simulink model "Project_lqr_control"  (R2025b)
settings: Solver=FixedStepDiscrete  StartTime=0.0  StopTime=inf  FixedStep=TS  RelTol=1e-3  EnableMultiTasking=on
values from neighbouring files (symbols this model uses):
  ES = -C2DEG*D2R    (= -0.00872664625997)    [NXT_Parameters.m]
  GS = GyroS*D2R    [NXT_Parameters.m]
  KLQR = [ 70.7107   73.7136 -108.1757  -16.8574]    [NXT_Parameters.m]    (also in Project_Jayce.m = lqr(A_b, B_b, Q, R))
  Rw = 0.021336    [NXT_Parameters.m]
  TS = 0.005    [NXT_Parameters.m]
libraries: arduinolib x3, simulink x1
settings Model: ExtModeTrigDuration=2  Creator=Sang  LastModifiedBy=jboar
settings SolverCC: AlgebraicLoopSolver=TrustRegion
settings DataIOCC: ReturnWorkspaceOutputs=off
settings OptimizationCC: MaxStackSize=64  EfficientTunableParamExpr=on
settings DebuggingCC: ParameterTunabilityLossMsg=error  UnconnectedInputMsg=warning  UnconnectedOutputMsg=warning  UnconnectedLineMsg=warning  ArithmeticOperatorsInVariantConditions=warning
settings HardwareCC: ProdBitPerInt=16.0  ProdBitPerPointer=16.0  ProdBitPerSizeT=16.0  ProdBitPerPtrDiffT=16.0  ProdLargestAtomicFloat=None  ProdWordSize=8.0  ProdHWDeviceType=Atmel->AVR
settings ModelReferenceCC: EnableRefExpFcnMdlSchedulingChecks=on
settings SFSimCC: SimUseLocalCustomCode=off  MATLABDynamicMemAlloc=off  CustomCodeUndefinedFunction=UseInterfaceOnly
settings RTWCC: SystemTargetFile=ert.tlc  HardwareBoard=Arduino Mega 2560  TemplateMakefile=ert_default_tmf  GenerateReport=on  RTWUseLocalCustomCode=off  Toolchain=Arduino AVR  BuildConfiguration=Faster Runs  IncludeHyperlinkInReport=on  LaunchReport=on  GenerateTraceInfo=on  GenerateTraceReport=on  GenerateTraceReportSl=on  GenerateTraceReportSf=on  GenerateTraceReportEml=on  GPUComputeCapability=3.5  Description=Embedded Coder
settings CodeAppCC: ForceParamTrailComments=on  IgnoreCustomStorageClasses=off  OperatorAnnotations=on  SimulinkDataObjDesc=on  SFDataObjDesc=on  MATLABFcnDesc=on  InsertBlockDesc=on  StateflowObjectComments=on  MATLABSourceComments=on
settings ERTTargetCC: InlinedParameterPlacement=Hierarchical  DynamicArrayContainerType=coder::array  MultiwordLength=2048.0  SupportContinuousTime=on  SupportVariableSizeSignals=on

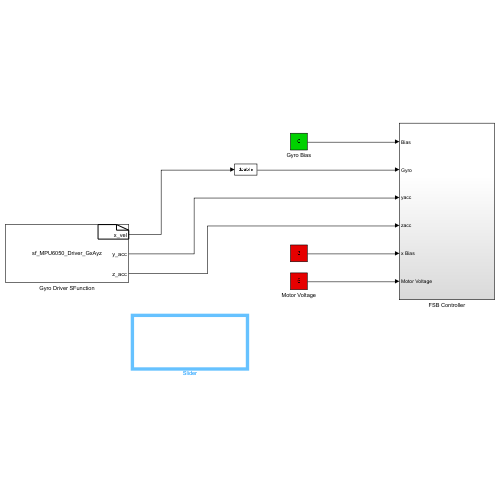
[thumbnail: Simulink's stored preview of the top-level diagram]
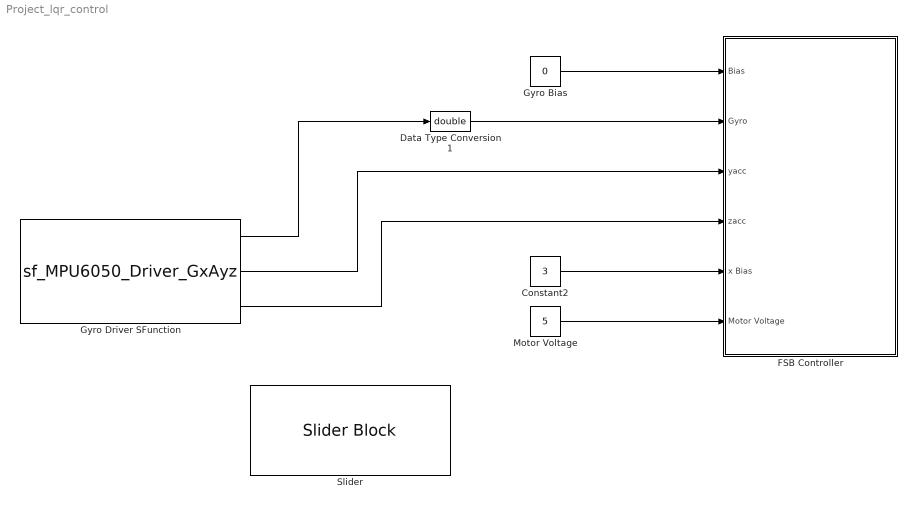
== system Project_lqr_control ==
  Constant2 : Constant  Value=3
  Data Type Conversion1 : DataTypeConversion  OutDataTypeStr=double  SaturateOnIntegerOverflow=off  RndMeth=Floor
  FSB Controller : Subsystem
  Gyro Bias : Constant  Value=0
  Gyro Driver SFunction : S-Function  InitFcn=try, set_param(gcb,'FunctionName','sf_MPU6050_Driver_GxAyz'), end  FunctionName=sf_MPU6050_Driver_GxAyz  SFunctionModules=sf_MPU6050_Driver_GxAyz_wrapper.cpp  SFunctionDeploymentMode=off  EnableBusSupport=off  mask(S-Function Builder){}
      mask help: Simulink:masks:SFunctionBuilder_MD
      mask init:
      | val = [[.9  0.75 0.75 1 1 .9 .9 1]',[1 1 0.75 0.75 .9 .9 1 .9]'];try , sys = get_param(gcb,'SfunBuilderFcnName');if isempty(sys), sys = get_param(gcb,'FunctionName'); end,catch, sys = get_param(gcb,'FunctionName'); end
      settings: CopyFcn=set_param(gcbh,'LinkStatus','none')  PreSaveFcn=try, set_param(gcb,'FunctionName','sf_MPU6050_Driver_GxAyz'), end  OpenFcn=sfunctionwizard(gcbh)
      mask Display:
      | plot(val(:,1),val(:,2))
      | disp(sys)
      | port_label('output',1,sprintf('%s', 'x\_vel'),'interpreter','tex')
      | port_label('output',2,sprintf('%s', 'y\_acc'),'interpreter','tex')
      | port_label('output',3,sprintf('%s', 'z\_acc'),'interpreter','tex')
  Motor Voltage : Constant  Value=5
  Slider : SliderBlock  ScaleMin=-20  ScaleMax=20
  wires:
  Gyro Driver SFunction/2 -> FSB Controller/3("yacc ")
  Gyro Driver SFunction/3 -> FSB Controller/4("zacc ")
  Gyro Bias/1 -> FSB Controller/1(Bias)
  Constant2/1 -> FSB Controller/5(x Bias)
  Motor Voltage/1 -> FSB Controller/6(Motor Voltage)
  Gyro Driver SFunction/1 -> Data Type Conversion1/1
  Data Type Conversion1/1 -> FSB Controller/2(Gyro)

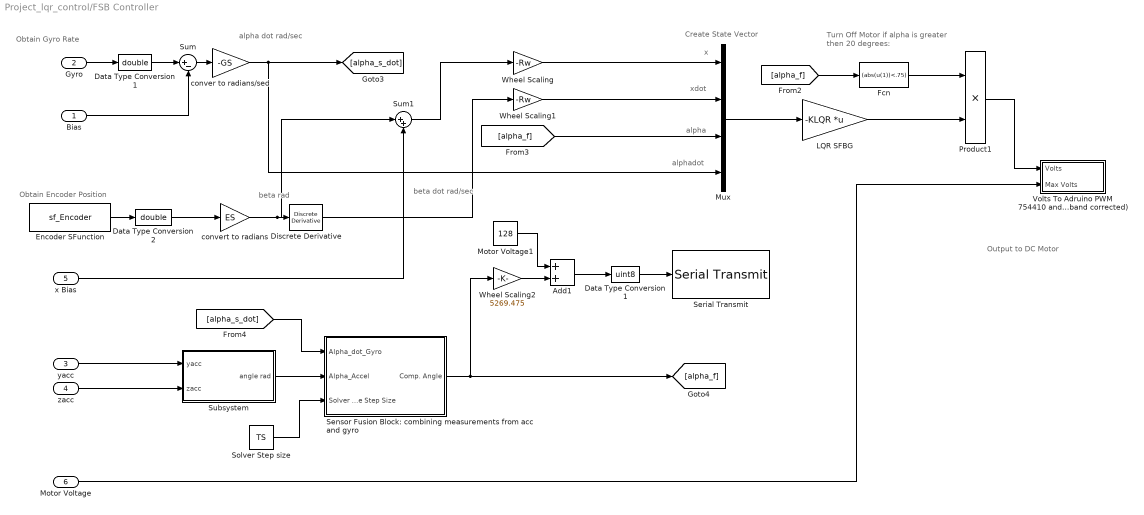
== system Project_lqr_control/FSB Controller ==
  note: Turn Off Motor if alpha is
      | greater then 20 degrees:
  note: Output to DC Motor
  note: Create State Vector
  note: Obtain Encoder Position
  note: Obtain Gyro Rate
  note: xdot
  note: x
  note: beta
      | rad
  note: alpha dot
      | rad/sec
  note: beta dot
      | rad/sec
  note: alpha
  note: alphadot
  Bias : Inport
  Gyro : Inport  Port=2
  "yacc " : Inport  Port=3
  "zacc " : Inport  Port=4
  x Bias : Inport  Port=5
  Motor Voltage : Inport  Port=6
  Add1 : Sum
  Data Type Conversion1 : DataTypeConversion  OutDataTypeStr=double  SaturateOnIntegerOverflow=off  RndMeth=Floor
  Data Type Conversion2 : DataTypeConversion  OutDataTypeStr=double  SaturateOnIntegerOverflow=off  RndMeth=Floor
  Data Type Conversion1 : DataTypeConversion  OutDataTypeStr=uint8  RndMeth=Nearest  SaturateOnIntegerOverflow=off
  Discrete Derivative : simulink/Discrete/Discrete Derivative  gainval=1.0  ICPrevScaledInput=0.0  OutMin=[]  OutMax=[]  OutDataType=fixdt(1, 16)  OutScaling=2^-10  DoSatur=off
  Encoder SFunction : S-Function  InitFcn=try, set_param(gcb,'FunctionName','sf_Encoder'), end  FunctionName=sf_Encoder  Parameters=uint8(0),uint8(18),uint8(19)  SFunctionModules=sf_Encoder_wrapper  SFunctionDeploymentMode=off  EnableBusSupport=off  mask(S-Function Builder){}
      mask init: same as Project_lqr_control/Gyro Driver SFunction
      settings: CopyFcn=set_param(gcbh,'LinkStatus','none')  PreSaveFcn=try, set_param(gcb,'FunctionName','sf_Encoder'), end  OpenFcn=sfunctionwizard(gcbh)
      mask Display: plot(val(:,1),val(:,2)),disp(sys), port_label('output',1,'pos')
  Fcn : Fcn  Expr=(abs(u(1))<.75)
  LQR SFBG : Gain  Gain=-KLQR  Multiplication=Matrix(K*u)
  Motor Voltage1 : Constant  Value=128
  Mux : Mux
  Product1 : Product  RndMeth=Zero
  Sensor Fusion Block: combining measurements from acc and gyro : Subsystem
  Serial Transmit : arduinolib/Serial Transmit  portNumber=2  sendmode=write  sendformat=Decimal  floatprecision=2  header=[]  terminator=[]  blockPlatform=arduino
  Solver Step size : Constant  Value=TS
  Subsystem : Subsystem
  Sum : Sum  Inputs=|+-
  Sum1 : Sum  Inputs=|++
  Volts To Adruino PWM 754410 and Motor1 (Deadband corrected) : Subsystem
  Wheel Scaling : Gain  Gain=-Rw
  Wheel Scaling1 : Gain  Gain=-Rw
  Wheel Scaling2 : Gain  Gain=5269.475
  conver to radians/sed : Gain  Gain=-GS
  convert to radians : Gain  Gain=ES  OutDataTypeStr=double
  wires:
  Bias/1 -> Sum/2
  Sum/1 -> conver to radians/sed/1
  convert to radians/1 -> Sum1/1, Discrete Derivative/1
  Data Type Conversion1/1 -> Sum/1
  Gyro/1 -> Data Type Conversion1/1
  [alpha_f] -> Fcn/1
  conver to radians/sed/1 -> [alpha_s_dot], Mux/4
  "yacc "/1 -> Subsystem/1(yacc)
  "zacc "/1 -> Subsystem/2(zacc)
  [alpha_f] -> Mux/3
  LQR SFBG/1 -> Product1/2
  Fcn/1 -> Product1/1
  Mux/1 -> LQR SFBG/1
  Wheel Scaling/1 -> Mux/1
  Subsystem/1(angle rad) -> Sensor Fusion Block: combining measurements from acc and gyro/2(Alpha_Accel)
  [alpha_s_dot] -> Sensor Fusion Block: combining measurements from acc and gyro/1(Alpha_dot_Gyro)
  Solver Step size/1 -> Sensor Fusion Block: combining measurements from acc and gyro/3(Solver Time Step Size)
  Sensor Fusion Block: combining measurements from acc and gyro/1(Comp. Angle) -> Wheel Scaling2/1, [alpha_f]
  Wheel Scaling1/1 -> Mux/2
  x Bias/1 -> Sum1/2
  Sum1/1 -> Wheel Scaling/1
  Encoder SFunction/1 -> Data Type Conversion2/1
  Data Type Conversion2/1 -> convert to radians/1
  Product1/1 -> Volts To Adruino PWM 754410 and Motor1 (Deadband corrected)/1(Volts)
  Motor Voltage/1 -> Volts To Adruino PWM 754410 and Motor1 (Deadband corrected)/2(Max Volts)
  Data Type Conversion1/1 -> Serial Transmit/1
  Add1/1 -> Data Type Conversion1/1
  Wheel Scaling2/1 -> Add1/2
  Motor Voltage1/1 -> Add1/1
  Discrete Derivative/1 -> Wheel Scaling1/1

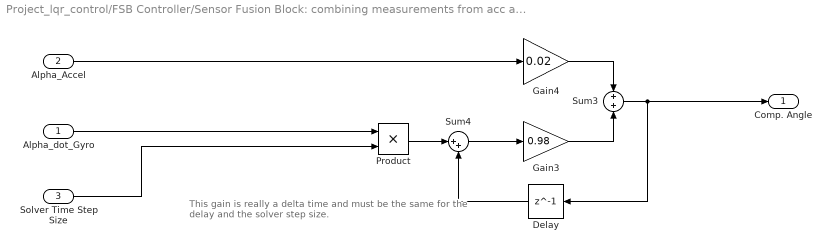
== system Project_lqr_control/FSB Controller/Sensor Fusion Block: combining measurements from acc and gyro ==
  note: This gain is really a delta time and must be the same for
      | the delay and the solver step size.
  Alpha_dot_Gyro : Inport
  Alpha_Accel : Inport  Port=2
  Solver Time Step Size : Inport  Port=3
  Delay : Delay  DelayLength=1  InitialCondition=0
  Gain3 : Gain  Gain=0.98
  Gain4 : Gain  Gain=0.02
  Product : Product
  Sum3 : Sum
  Sum4 : Sum  Inputs=|++
  Comp. Angle : Outport  VectorParamsAs1DForOutWhenUnconnected=off
  wires:
  Gain3/1 -> Sum3/2
  Gain4/1 -> Sum3/1
  Sum3/1 -> Comp. Angle/1, Delay/1
  Sum4/1 -> Gain3/1
  Delay/1 -> Sum4/2
  Product/1 -> Sum4/1
  Alpha_Accel/1 -> Gain4/1
  Alpha_dot_Gyro/1 -> Product/1
  Solver Time Step Size/1 -> Product/2

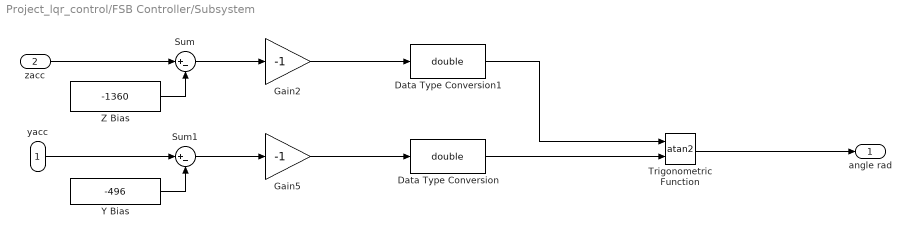
== system Project_lqr_control/FSB Controller/Subsystem ==
  yacc : Inport
  zacc : Inport  Port=2
  Data Type Conversion : DataTypeConversion  OutDataTypeStr=double  SaturateOnIntegerOverflow=off  RndMeth=Floor
  Data Type Conversion1 : DataTypeConversion  OutDataTypeStr=double  SaturateOnIntegerOverflow=off  RndMeth=Floor
  Gain2 : Gain  Gain=-1
  Gain5 : Gain  Gain=-1
  Sum : Sum  Inputs=|+-
  Sum1 : Sum  Inputs=|+-
  Trigonometric Function : Trigonometry  Operator=atan2
  Y Bias : Constant  Value=-496
  Z Bias : Constant  Value=-1360
  angle rad : Outport  VectorParamsAs1DForOutWhenUnconnected=off
  wires:
  Z Bias/1 -> Sum/2
  Y Bias/1 -> Sum1/2
  Trigonometric Function/1 -> angle rad/1
  Data Type Conversion1/1 -> Trigonometric Function/1
  Data Type Conversion/1 -> Trigonometric Function/2
  zacc/1 -> Sum/1
  yacc/1 -> Sum1/1
  Gain2/1 -> Data Type Conversion1/1
  Sum/1 -> Gain2/1
  Sum1/1 -> Gain5/1
  Gain5/1 -> Data Type Conversion/1

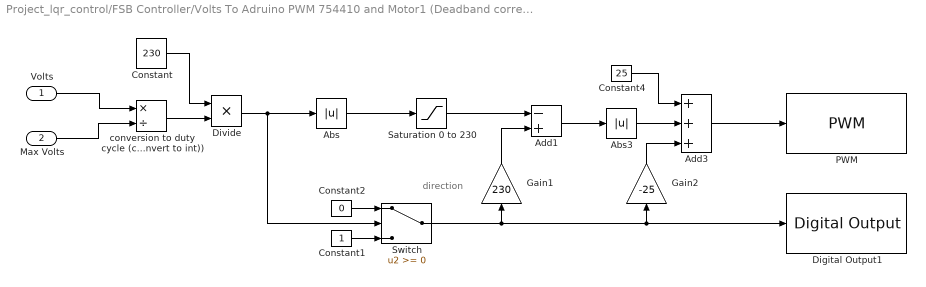
== system Project_lqr_control/FSB Controller/Volts To Adruino PWM 754410 and Motor1 (Deadband corrected) ==
  note: direction
  Volts : Inport
  Max Volts : Inport  Port=2
  Abs : Abs  SaturateOnIntegerOverflow=off
  Abs3 : Abs  SaturateOnIntegerOverflow=off
  Add1 : Sum  Inputs=-+
  Add3 : Sum  Inputs=+++
  Constant : Constant  Value=230
  Constant1 : Constant
  Constant2 : Constant  Value=0
  Constant4 : Constant  Value=25
  Digital Output1 : arduinolib/Digital Output  pinNumber=8  Direction=output  blockPlatform=arduino
  Divide : Product  Inputs=**
  Gain1 : Gain  Gain=230
  Gain2 : Gain  Gain=-25
  PWM : arduinolib/PWM  pinNumber=6  frequencyType=Default  desiredFrequency=490.2  achievableFrequency=490.2
  Saturation 0 to 230 : Saturate  UpperLimit=230  LowerLimit=0
  Switch : Switch  SaturateOnIntegerOverflow=off  InputSameDT=off
  conversion to duty cycle (convert to int)) : Product  Inputs=*/  OutDataTypeStr=double
  wires:
  Abs/1 -> Saturation 0 to 230/1
  Saturation 0 to 230/1 -> Add1/1
  Add1/1 -> Abs3/1
  Gain1/1 -> Add1/2
  Constant1/1 -> Switch/3
  Constant2/1 -> Switch/1
  Switch/1 -> Gain1/1, Gain2/1, Digital Output1/1
  Abs3/1 -> Add3/2
  Add3/1 -> PWM/1
  Constant4/1 -> Add3/1
  Volts/1 -> conversion to duty cycle (convert to int))/1
  Max Volts/1 -> conversion to duty cycle (convert to int))/2
  Divide/1 -> Switch/2, Abs/1
  conversion to duty cycle (convert to int))/1 -> Divide/2
  Constant/1 -> Divide/1
  Gain2/1 -> Add3/3
